simulink model "RailP_VDSync"  (R2016b)
settings: configuration reference "CodeGenConfigSet" (kept outside this file)
settings Model: Creator=zhoutinglin  LastModifiedBy=zhoutinglin
settings ConfigSetRef: SourceLocation=Base Workspace

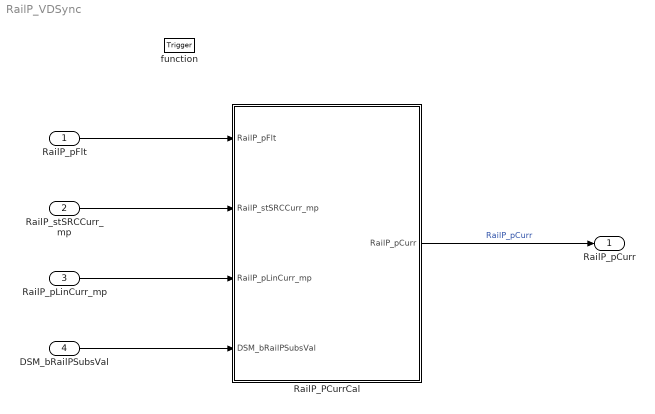
== system RailP_VDSync ==
  RailP_pFlt : Inport  Tag=bar  Description=Maximum rail pressure of the last 10 sampling cycle  OutMin=0  OutMax=2500  OutDataTypeStr=RailPressure_bar
  RailP_stSRCCurr_mp : Inport  Description=Maximum SRC default value  Port=2  OutMin=0  OutMax=1  OutDataTypeStr=boolean
  RailP_pLinCurr_mp : Inport  Tag=bar  Description=Linearisation value current rail pressure  Port=3  OutMin=0  OutMax=2500  OutDataTypeStr=RailPressure_bar
  DSM_bRailPSubsVal : Inport  Description=Status of FId_RailPSubsVal  Port=4  OutMin=0  OutMax=1  OutDataTypeStr=boolean
  function : TriggerPort  TriggerType=function-call  VariantControl=Variant
  RailP_PCurrCal : Subsystem
  RailP_pCurr : Outport  Tag=bar  Description=Current fuel pressure  OutMin=0  OutMax=2500  OutDataTypeStr=RailPressure_bar
  wires:
  RailP_PCurrCal/1(RailP_pCurr) -> RailP_pCurr/1  "RailP_pCurr"
  DSM_bRailPSubsVal/1 -> RailP_PCurrCal/4(DSM_bRailPSubsVal)
  RailP_stSRCCurr_mp/1 -> RailP_PCurrCal/2(RailP_stSRCCurr_mp)
  RailP_pFlt/1 -> RailP_PCurrCal/1(RailP_pFlt)
  RailP_pLinCurr_mp/1 -> RailP_PCurrCal/3(RailP_pLinCurr_mp)

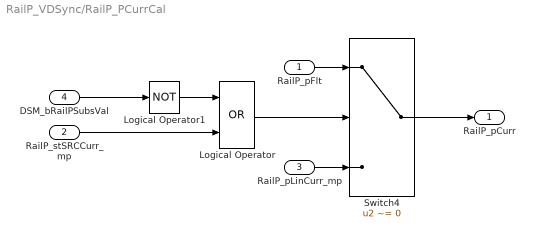
== system RailP_VDSync/RailP_PCurrCal ==
  RailP_pFlt : Inport  Tag=bar  Description=Fuel pressure  OutMin=0  OutMax=2500  OutDataTypeStr=RailPressure_bar
  RailP_stSRCCurr_mp : Inport  Description=status of SRC  Port=2  OutMin=0  OutMax=1  OutDataTypeStr=boolean
  RailP_pLinCurr_mp : Inport  Tag=bar  Description=current pressure  Port=3  OutMin=0  OutMax=2500  OutDataTypeStr=RailPressure_bar
  DSM_bRailPSubsVal : Inport  Description=status of FId_RailPSubsVal  Port=4  OutMin=0  OutMax=1  OutDataTypeStr=boolean
  Logical Operator : Logic  Operator=OR  OutDataTypeStr=boolean
  Logical Operator1 : Logic  Operator=NOT  AllPortsSameDT=off  OutDataTypeStr=boolean
  Switch4 : Switch  Criteria=u2 ~= 0  InputSameDT=on
  RailP_pCurr : Outport  Tag=bar  Description=Current fuel pressure  OutMin=0  OutMax=2500  OutDataTypeStr=RailPressure_bar
  wires:
  RailP_pLinCurr_mp/1 -> Switch4/3
  RailP_stSRCCurr_mp/1 -> Logical Operator/2
  DSM_bRailPSubsVal/1 -> Logical Operator1/1
  Logical Operator1/1 -> Logical Operator/1
  Switch4/1 -> RailP_pCurr/1
  Logical Operator/1 -> Switch4/2
  RailP_pFlt/1 -> Switch4/1
